simulink model "pendulum_sim_in"  (R2016a)
settings: Solver=ode45  StartTime=0.0  StopTime=300  RelTol=1e-3
undefined symbols (not defined in the file or in its folder): P
libraries: cstblocks x2
settings Model: Creator=beard  LastModifiedBy=beard
settings DataIOCC: LimitDataPoints=on  SaveFormat=Array  SignalLoggingSaveFormat=ModelDataLogs
settings OptimizationCC: ExpressionDepthLimit=2147483647  InitFltsAndDblsToZero=on
settings DebuggingCC: UnderspecifiedInitializationDetection=Classic  MergeDetectMultiDrivingBlocksExec=none  SolverPrmCheckMsg=warning  FcnCallInpInsideContextMsg=UseLocalSettings  StateNameClashWarn=warning
settings HardwareCC: ProdBitPerPointer=32  ProdLargestAtomicFloat=None  ProdIntDivRoundTo=Undefined  ProdEndianess=Unspecified  ProdWordSize=32  ProdHWDeviceType=32-bit Generic
settings ModelReferenceCC: PropagateSignalLabelsOutOfModel=off
settings GRTTargetCC: CombineOutputUpdateFcns=off  GRTInterface=on
settings ConfigComp: CovModelRefEnable=Off

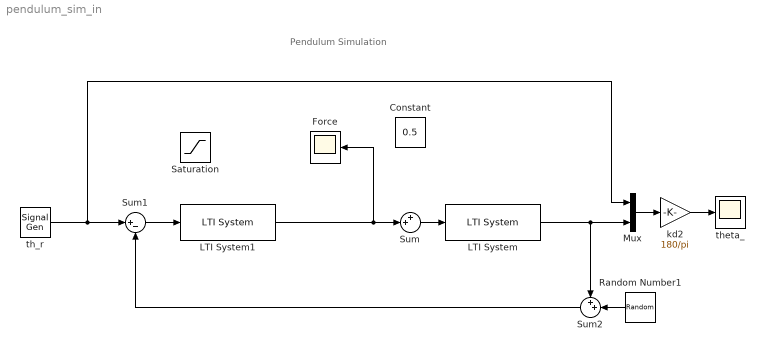
== system pendulum_sim_in ==
  note: Pendulum Simulation
  Constant : Constant  Value=0.5
  Force : Scope
  LTI System : cstblocks/LTI System  sys=P_in  IC=[]
  LTI System1 : cstblocks/LTI System  sys=C_in  IC=[]
  Mux : Mux  Inputs=2
  Random Number1 : RandomNumber  Variance=.001^2  SampleTime=P.Ts
  Saturation : Saturate  UpperLimit=P.F_max  LowerLimit=-P.F_max
  Sum : Sum  Inputs=++|
  Sum1 : Sum  Inputs=|+-
  Sum2 : Sum  Inputs=++|
  kd2 : Gain  Gain=180/pi
  th_r : SignalGenerator  WaveForm=square  Amplitude=2*pi/180  Frequency=.02
  theta_ : Scope
  wires:
  kd2/1 -> theta_/1
  Sum/1 -> LTI System/1
  Sum2/1 -> Sum1/2
  LTI System/1 -> Mux/2, Sum2/1
  Random Number1/1 -> Sum2/2
  Mux/1 -> kd2/1
  Sum1/1 -> LTI System1/1
  th_r/1 -> Mux/1, Sum1/1
  LTI System1/1 -> Force/1, Sum/2
